simulink model "gainSchedExample_nonlinPlant_linearCntr"  (R2020b)
settings: Solver=VariableStepAuto  StartTime=0.0  StopTime=10.0  MinStep=TSim/5000  RelTol=1e-3
values from neighbouring files (symbols this model uses):
  cntr =     [cntrDesign_1.mat]    (also in cntrDesign_2.mat)
  initVal = 1    [Run_AcademicExample.m]
  refVal = 1.5    [Run_AcademicExample.m]
  tStep = 3.5    [Run_AcademicExample.m]
  umax = 8    [Design_ControllerObserverAndAW.m]    (also in Run_AcademicExample.m = 800)
  xInit = cntr.xAP_1    [Design_ControllerObserverAndAW.m]    (also in Run_AcademicExample.m)
undefined symbols (not defined in the file or in its folder): system
settings Model: Creator=Kefferpuetz  LastModifiedBy=Kefferpuetz

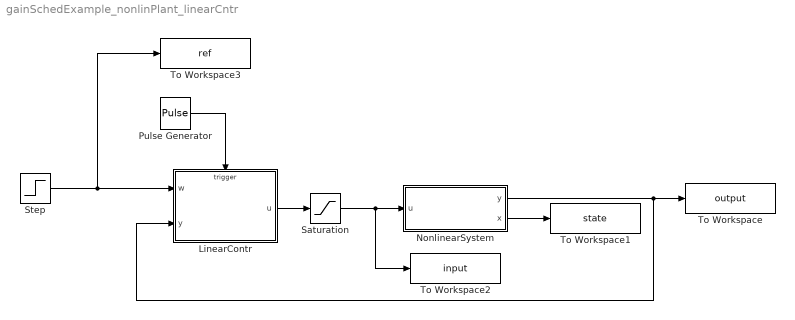
== system gainSchedExample_nonlinPlant_linearCntr ==
  LinearContr : Subsystem
  NonlinearSystem : Subsystem
  Pulse Generator : DiscretePulseGenerator  PulseType=Time based  Period=cntr.TS  PulseWidth=50
  Saturation : Saturate  UpperLimit=umax  LowerLimit=-umax
  Step : Step  Time=tStep  Before=initVal  After=refVal  SampleTime=0
  To Workspace : ToWorkspace  VariableName=output  SaveFormat=Structure With Time  SampleTime=-1
  To Workspace1 : ToWorkspace  VariableName=state  SaveFormat=Structure With Time  SampleTime=-1
  To Workspace2 : ToWorkspace  VariableName=input  SaveFormat=Structure With Time  SampleTime=-1
  To Workspace3 : ToWorkspace  VariableName=ref  SaveFormat=Structure With Time  SampleTime=-1
  wires:
  NonlinearSystem/2(x) -> To Workspace1/1
  NonlinearSystem/1(y) -> To Workspace/1, LinearContr/2(y)
  LinearContr/1(u) -> Saturation/1
  Saturation/1 -> To Workspace2/1, NonlinearSystem/1(u)
  Step/1 -> To Workspace3/1, LinearContr/1(w)
  Pulse Generator/1 -> LinearContr/Trigger

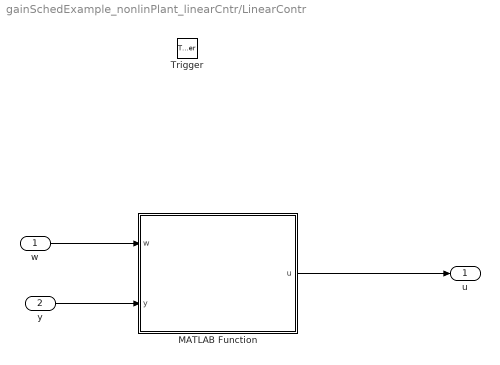
== system gainSchedExample_nonlinPlant_linearCntr/LinearContr ==
  w : Inport
  y : Inport  Port=2
  Trigger : TriggerPort  VariantControl=Variant  PortDimensions=1
  MATLAB Function : MATLAB Function  TreatAsAtomicUnit=on
  u : Outport
  wires:
  MATLAB Function/1(u) -> u/1
  y/1 -> MATLAB Function/2(y)
  w/1 -> MATLAB Function/1(w)

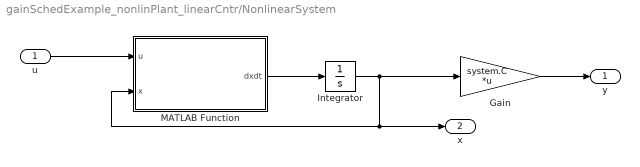
== system gainSchedExample_nonlinPlant_linearCntr/NonlinearSystem ==
  u : Inport
  Gain : Gain  Gain=system.C  Multiplication=Matrix(K*u) (u vector)
  Integrator : Integrator  InitialCondition=xInit
  MATLAB Function : MATLAB Function  TreatAsAtomicUnit=on
  y : Outport
  x : Outport  Port=2
  wires:
  Gain/1 -> y/1
  Integrator/1 -> Gain/1, MATLAB Function/2(x), x/1
  MATLAB Function/1(dxdt) -> Integrator/1
  u/1 -> MATLAB Function/1(u)

== matlab function gainSchedExample_nonlinPlant_linearCntr/LinearContr/MATLAB Function ==
  data: w input; y input; u output; cntr parameter
function u  = linearCntr(w, y,  cntr)
  % This function implements a discretized version of a pure linear
  % controller applied near operating point cntr.xAP of the nonlinear
  % plant.
  % 
  % Author: Klaus Kefferpütz, University of Applied Sciences Augsburg 2021
  % email: klaus.kefferpuetz@hs-augsburg.de
  persistent xI;
  persistent xEst;
  
  if(isempty(xI))
     xI = 0;
     xEst = cntr.initState; 
  end
  
  TS = cntr.TS;
  yAP = cntr.xAP(1);
  
  % compute controller inputs
  delta_y = y-yAP;

  % Compute PI-state space control law
  u = cntr.Kp*(w-y)+cntr.Ki*xI-cntr.K*xEst+cntr.uAP;
  
  % update integrator state of PI state space controller
  xI = xI+TS*(w-y);
  
  % update linear observer
  yEst     = cntr.C*xEst;
  xEst_kP  = xEst + TS*( cntr.A*xEst+cntr.B*(u-cntr.uAP)+cntr.L*(delta_y-yEst));  
  xEst     = xEst_kP;

== matlab function gainSchedExample_nonlinPlant_linearCntr/NonlinearSystem/MATLAB Function ==
  data: u input; x input; dxdt output
function dxdt  = fcn(u, x)
    dxdt = zeros(2,1);    

    
   
    dxdt(1) = x(2);
    dxdt(2) = x(1)*(1-x(2))+u;
